simulink model "Attitudesim"  (R2023a)
settings: Solver=FixedStepAuto  StartTime=0.0  StopTime=tf  FixedStep=tstep  RelTol=1e-3  EnableMultiTasking=on
values from neighbouring files (symbols this model uses):
  C = [1 0 0 0 0 0;     0 1 0 0 0 0;     0 0 1 0 0 0]    [Attitude.m]    (also in Translational.m = eye(6))
  Co = [C;0 0 0 1 0 0;     0 0 0 0 1 0;     0 0 0 0 0 1]    [Attitude.m]
  I = [Ixx,Iyy,Izz]    [Attitude.m]
  K = -inv(R)*Bbar'*P    [Attitude.m]
  L = Pltr*Co'*inv(Ro)    [Attitude.m]    (also in Translational.m = Pltr*C'*inv(Ro))
  ref = [pi/18 pi/32 0]    [Attitude.m]    (also in Translational.m = [0 0 -2]; main.m = [1;1;-2])
  tstep = 0.001    [Attitude.m]    (also in Translational.m; main.m)
  xi = [0; pi/6; 0; 0; 0; 0]    [Attitude.m]    (also in Translational.m = [0; 0; 0; 0; 0; 0])
libraries: simulink x1
settings Model: Creator=Nathan Dablain  LastModifiedBy=Nathan Dablain

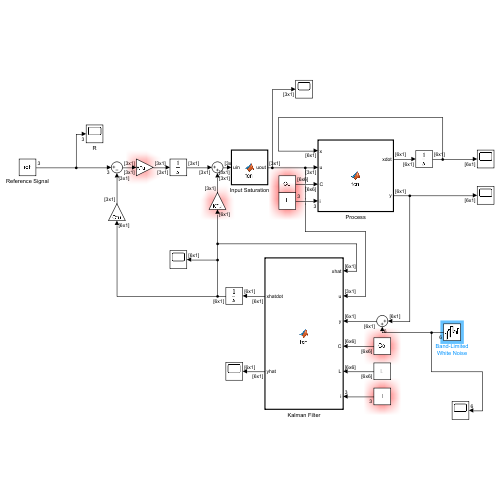
[thumbnail: Simulink's stored preview of the top-level diagram]
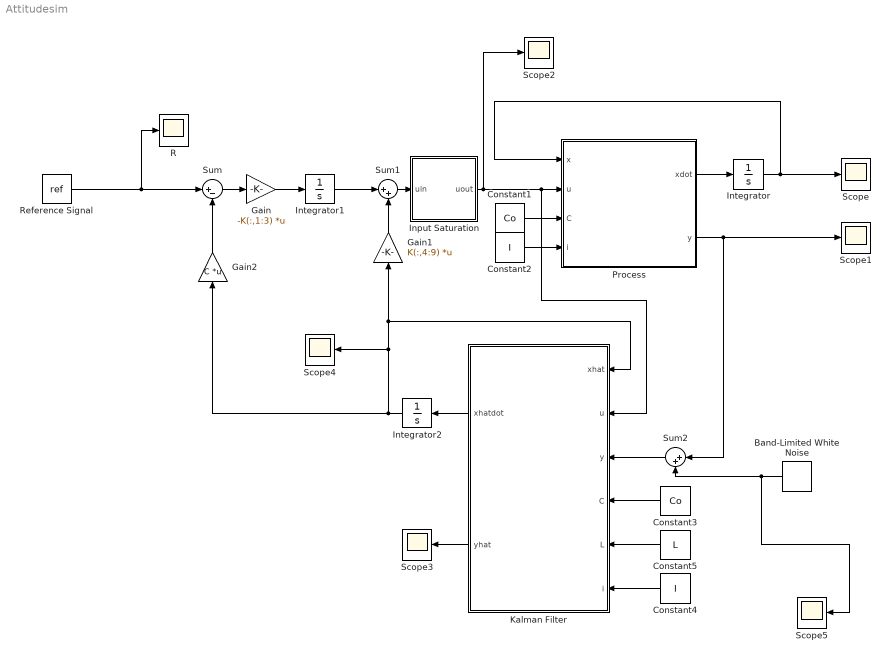
== system Attitudesim ==
  Band-Limited White Noise : simulink/Sources/Band-Limited White Noise  Cov=[5e-6 5e-6 5e-6 1e-6 1e-6 1e-6]  Ts=tstep  seed=[23341]
  Constant1 : Constant  Value=Co
  Constant2 : Constant  Value=I
  Constant3 : Constant  Value=Co
  Constant4 : Constant  Value=I
  Constant5 : Constant  Value=L
  Gain : Gain  Gain=-K(:,1:3)  Multiplication=Matrix(K*u)
  Gain1 : Gain  Gain=K(:,4:9)  Multiplication=Matrix(K*u)
  Gain2 : Gain  Gain=C  Multiplication=Matrix(K*u)
  Input Saturation : MATLAB Function  TreatAsAtomicUnit=on
  Integrator : Integrator  InitialCondition=xi
  Integrator1 : Integrator  InitialCondition=zeros(3,1)
  Integrator2 : Integrator  InitialCondition=zeros(6,1)
  Kalman Filter : MATLAB Function  TreatAsAtomicUnit=on
  Process : MATLAB Function  TreatAsAtomicUnit=on
  R : Scope
  Reference Signal : Constant  Value=ref
  Scope{,1..5} (6 alike) : Scope
  Sum : Sum  Inputs=|+-
  Sum1 : Sum  Inputs=|++
  Sum2 : Sum  Inputs=|++
  wires:
  Process/1(xdot) -> Integrator/1
  Integrator/1 -> Process/1(x), Scope/1
  Process/2(y) -> Sum2/1, Scope1/1
  Constant1/1 -> Process/3(C)
  Integrator1/1 -> Sum1/1
  Sum/1 -> Gain/1
  Gain1/1 -> Sum1/2
  Reference Signal/1 -> R/1, Sum/1
  Sum1/1 -> Input Saturation/1(uin)
  Input Saturation/1(uout) -> Scope2/1, Kalman Filter/2(u), Process/2(u)
  Gain/1 -> Integrator1/1
  Constant2/1 -> Process/4(i)
  Kalman Filter/1(xhatdot) -> Integrator2/1
  Integrator2/1 -> Gain1/1, Kalman Filter/1(xhat), Scope4/1, Gain2/1
  Sum2/1 -> Kalman Filter/3(y)
  Band-Limited White Noise/1 -> Scope5/1, Sum2/2
  Constant3/1 -> Kalman Filter/4(C)
  Constant4/1 -> Kalman Filter/6(i)
  Gain2/1 -> Sum/2
  Kalman Filter/2(yhat) -> Scope3/1
  Constant5/1 -> Kalman Filter/5(L)

== matlab function Attitudesim/Kalman Filter ==
  data: xhat input; xhatdot output; u input; y input; yhat output; C input; L input; i input
function [xhatdot,yhat] = fcn(xhat,u,y,C,L,i)
I = diag([i(1) i(2) i(3)]);
yhat = C*xhat;
xhatdot = [[1 sin(xhat(1))*tan(xhat(2)) cos(xhat(1))*tan(xhat(2));...
    0 cos(xhat(1)) -sin(xhat(1));...
    0 sin(xhat(1))*sec(xhat(2)) cos(xhat(1))*sec(xhat(2))]*xhat(4:6);...
    I\(u - cross(xhat(4:6),I*xhat(4:6)))] + L*(y-yhat);
end

== matlab function Attitudesim/Process ==
  data: x input; xdot output; u input; y output; C input; i input
function [xdot,y] = fcn(x,u,C,i)
I = [i(1)+0.01 -0.001 -0.001;...
    -0.001 i(2)-0.01 -0.001;...
    -0.001 -0.001 i(3)+0.02];
xdot = [[1 sin(x(1))*tan(x(2)) cos(x(1))*tan(x(2));...
    0 cos(x(1)) -sin(x(1));...
    0 sin(x(1))*sec(x(2)) cos(x(1))*sec(x(2))]*x(4:6);...
    I\(u - cross(x(4:6),I*x(4:6)))];
y = C*x;
end

== matlab function Attitudesim/Input Saturation ==
  data: uin input; uout output
function uout = fcn(uin)
uout = uin;
max_thrust = 30; % N
max_torque = max_thrust*0.2; % N-m
for i = 1:3
    if uin(i) > max_torque
        uout(i) = max_torque;
    elseif uin(i) < -max_torque
        uout(i) = -max_torque;
    end
end
end
